simulink model "manualControl"  (R2019a)
settings: Solver=FixedStepDiscrete  StartTime=0.0  StopTime=60  FixedStep=0.1  RelTol=1e-3  EnableMultiTasking=on
model workspace (MAT data in the model file):
  SL_ROS_VariableLengthArrays_MaxSizes.CommonInfo.ArrayTruncateAction = 'EmitWarning'
  SL_ROS_VariableLengthArrays_MaxSizes.MsgTypeMap = containers.Map
  SL_ROS_VariableLengthArrays_MaxSizes.MsgTypeMap.serialization.keys = {'sensor_msgs/Image', 'sensor_msgs/LaserScan'}
  SL_ROS_VariableLengthArrays_MaxSizes.MsgTypeMap.serialization.values{1}(1).PropertyName = 'Data'
  SL_ROS_VariableLengthArrays_MaxSizes.MsgTypeMap.serialization.values{1}(1).DataType = 'uint8'
  SL_ROS_VariableLengthArrays_MaxSizes.MsgTypeMap.serialization.values{1}(1).MaxLength = 691200
  SL_ROS_VariableLengthArrays_MaxSizes.MsgTypeMap.serialization.values{1}(2).PropertyName = 'Encoding'
  SL_ROS_VariableLengthArrays_MaxSizes.MsgTypeMap.serialization.values{1}(2).DataType = 'uint8'
  SL_ROS_VariableLengthArrays_MaxSizes.MsgTypeMap.serialization.values{1}(2).MaxLength = 128
  SL_ROS_VariableLengthArrays_MaxSizes.MsgTypeMap.serialization.values{2}(1).PropertyName = 'Intensities'
  SL_ROS_VariableLengthArrays_MaxSizes.MsgTypeMap.serialization.values{2}(1).DataType = 'single'
  SL_ROS_VariableLengthArrays_MaxSizes.MsgTypeMap.serialization.values{2}(1).MaxLength = 1081
  SL_ROS_VariableLengthArrays_MaxSizes.MsgTypeMap.serialization.values{2}(2).PropertyName = 'Ranges'
  SL_ROS_VariableLengthArrays_MaxSizes.MsgTypeMap.serialization.values{2}(2).DataType = 'single'
  SL_ROS_VariableLengthArrays_MaxSizes.MsgTypeMap.serialization.values{2}(2).MaxLength = 1081
  SL_ROS_VariableLengthArrays_MaxSizes.MsgTypeMap.serialization.uniformity = 0
  SL_ROS_VariableLengthArrays_MaxSizes.MsgTypeMap.serialization.keyType = 'char'
  SL_ROS_VariableLengthArrays_MaxSizes.MsgTypeMap.serialization.valueType = 'any'
undefined symbols (not defined in the file or in its folder): Angular, d, dfod, DiscIntNeverNeededParam, gray, ioKd, ioKi, ioKp, Kd, Kp, Linear
libraries: robotlib x6, simulink x2, aerolibanimutils x1
settings Model: Creator=The MathWorks, Inc.  LastModifiedBy=standard
settings DataIOCC: LimitDataPoints=on  SaveFormat=Array  ReturnWorkspaceOutputs=off
settings OptimizationCC: LifeSpan=Inf  MaxStackSize=64
settings DebuggingCC: SolverPrmCheckMsg=warning  SFUnexpectedBacktrackingDiag=warning  SFNoUnconditionalDefaultTransitionDiag=warning  SFExecutionAtInitializationDiag=none  ArithmeticOperatorsInVariantConditions=warning
settings HardwareCC: ProdBitPerPointer=32  ProdBitPerSizeT=32  ProdBitPerPtrDiffT=32  ProdLargestAtomicFloat=None  ProdIntDivRoundTo=Undefined  ProdEndianess=Unspecified  ProdWordSize=32  ProdHWDeviceType=Generic->Unspecified (assume 32-bit Generic)  UseEmbeddedCoderFeatures=off
settings ModelReferenceCC: PropagateSignalLabelsOutOfModel=off
settings SFSimCC: SimUseLocalCustomCode=off
settings RTWCC: SystemTargetFile=ert.tlc  HardwareBoard=Robot Operating System (ROS)  TLCOptions=-aInlineSetEventsForThisBaseRateFcn=TLC_FALSE -aSuppressMultiTaskScheduler=TLC_FALSE -aRateBasedStepFcn=0  TemplateMakefile=ert_default_tmf  RTWUseLocalCustomCode=off  Toolchain=Catkin  TargetLang=C++
settings CodeAppCC: StateflowObjectComments=on
settings ERTTargetCC: MultiwordLength=2048  ERTCustomFileBanners=off  SupportContinuousTime=on  SupportNonInlinedSFcns=on  RemoveResetFunc=off  SupportVariableSizeSignals=on  ModelStepFunctionPrototypeControlCompliant=off  ConvertIfToSwitch=off  SuppressUnreachableDefaultCases=off
settings ConfigComp: CovMetricSettings=dw  CovHtmlReporting=on  CovSaveCumulativeToWorkspaceVar=on  CovSaveSingleToWorkspaceVar=on  CovExternalEMLEnable=off  CovSFcnEnable=off

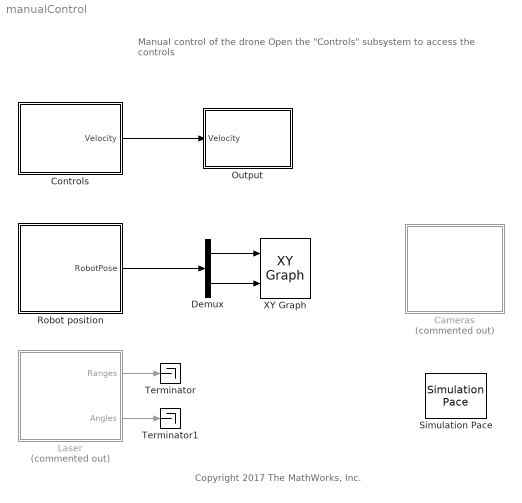
== system manualControl ==
  note: Manual control of the drone
      | Open the "Controls" subsystem to access the controls
  note: Copyright 2017 The MathWorks, Inc.
  Cameras : Subsystem  Commented=on
  Controls : Subsystem
  Demux : Demux  Outputs=2
  Laser : Subsystem  Commented=on
  Output : Subsystem
  Robot position : Subsystem
  Simulation Pace : aerolibanimutils/Simulation Pace  SimulationPace=1  SleepMode=MATLAB Thread  OutputPaceError=off  SampleTime=-1
  Terminator : Terminator
  Terminator1 : Terminator
  XY Graph : simulink/Sinks/XY Graph  xmin=-10  xmax=30  ymin=-10  ymax=10  st=-1
  wires:
  Controls/1(Velocity) -> Output/1(Velocity)
  Robot position/1(RobotPose) -> Demux/1
  Demux/1 -> XY Graph/1
  Demux/2 -> XY Graph/2
  Laser/1(Ranges) -> Terminator/1
  Laser/2(Angles) -> Terminator1/1

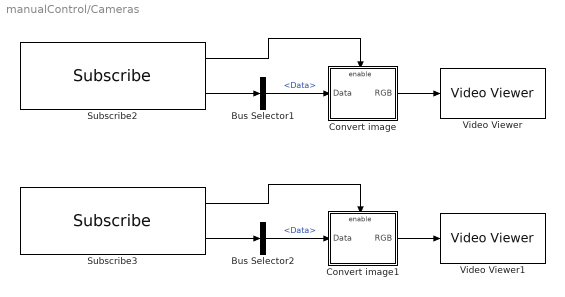
== system manualControl/Cameras ==
  Bus Selector1 : BusSelector  DialogController=Simulink.DDGSource_BusSelector  OutputSignals=Data
  Bus Selector2 : BusSelector  DialogController=Simulink.DDGSource_BusSelector  OutputSignals=Data
  Convert image : Subsystem
  Convert image1 : Subsystem
  Subscribe2 : robotlib/Subscribe  topicSource=Select from ROS network  topic=/quadrotor_1/front/image_raw  messageType=sensor_msgs/Image  sampleTime=-1  messageQueueLength=51
      settings: SourceProductBaseCode=RO
  Subscribe3 : robotlib/Subscribe  topicSource=Select from ROS network  topic=/quadrotor_1/bottom/image_raw  messageType=sensor_msgs/Image  sampleTime=-1  messageQueueLength=51
      settings: SourceProductBaseCode=RO
  Video Viewer : VideoViewer  colormapValue=gray(256)  FigPos=[672 404 609 271.6]
  Video Viewer1 : VideoViewer  colormapValue=gray(256)  FigPos=[671 757 610 376]
  wires:
  Subscribe2/1 -> Convert image/Enable
  Convert image1/1(RGB) -> Video Viewer1/1
  Subscribe3/2 -> Bus Selector2/1
  Subscribe2/2 -> Bus Selector1/1
  Bus Selector1/1 -> Convert image/1(Data)  "<Data>"
  Bus Selector2/1 -> Convert image1/1(Data)  "<Data>"
  Subscribe3/1 -> Convert image1/Enable
  Convert image/1(RGB) -> Video Viewer/1

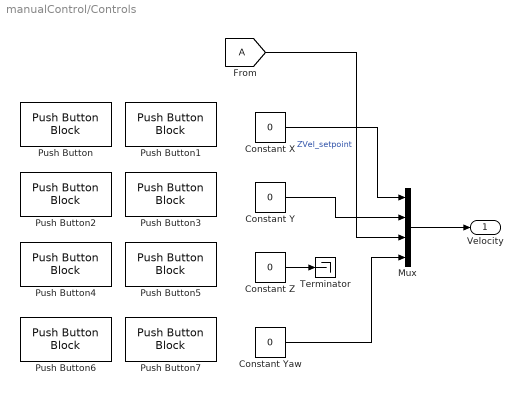
== system manualControl/Controls ==
  Constant X : Constant  Value=0
  Constant Y : Constant  Value=0
  Constant Yaw : Constant  Value=0
  Constant Z : Constant  Value=0
  Mux : Mux
  Push Button : PushButtonBlock  LabelPosition=Top  ButtonText=Backward  OnValue=-1
  Push Button1 : PushButtonBlock  LabelPosition=Top  ButtonText=Forward
  Push Button2 : PushButtonBlock  LabelPosition=Top  ButtonText=Left
  Push Button3 : PushButtonBlock  LabelPosition=Top  ButtonText=Right  OnValue=-1
  Push Button4 : PushButtonBlock  LabelPosition=Top  ButtonText=Down  OnValue=-1
  Push Button5 : PushButtonBlock  LabelPosition=Top  ButtonText=Up
  Push Button6 : PushButtonBlock  LabelPosition=Top  ButtonText=Counterclockwise
  Push Button7 : PushButtonBlock  LabelPosition=Top  ButtonText=Clockwise  OnValue=-1
  Terminator : Terminator
  Velocity : Outport
  wires:
  Mux/1 -> Velocity/1
  Constant Y/1 -> Mux/2
  Constant X/1 -> Mux/1
  [A] -> Mux/3  "ZVel_setpoint"
  Constant Yaw/1 -> Mux/4
  Constant Z/1 -> Terminator/1

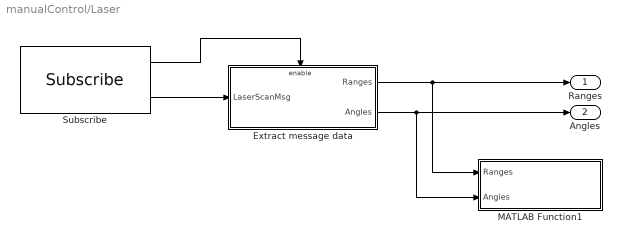
== system manualControl/Laser ==
  Extract message data : Subsystem
  MATLAB Function1 : MATLAB Function  TreatAsAtomicUnit=on
  Subscribe : robotlib/Subscribe  topicSource=Select from ROS network  topic=/quadrotor_1/scan  messageType=sensor_msgs/LaserScan  sampleTime=-1  messageQueueLength=1
      settings: SourceProductBaseCode=RO
  Ranges : Outport
  Angles : Outport  Port=2
  wires:
  Subscribe/1 -> Extract message data/Enable
  Extract message data/2(Angles) -> Angles/1, MATLAB Function1/2(Angles)
  Subscribe/2 -> Extract message data/1(LaserScanMsg)
  Extract message data/1(Ranges) -> Ranges/1, MATLAB Function1/1(Ranges)

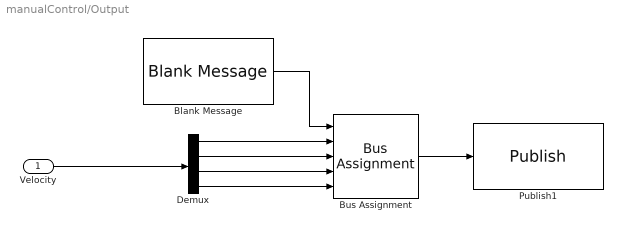
== system manualControl/Output ==
  Velocity : Inport
  Blank Message : robotlib/Blank Message  messageClass=Message  entityType=geometry_msgs/Twist  messageType=geometry_msgs/Twist  SampleTime=0
      settings: SourceProductBaseCode=RO
  Bus Assignment : BusAssignment  DialogController=Simulink.DDGSource_BusAssignment  AssignedSignals=Linear.X,Linear.Y,Linear.Z,Angular.Z
  Demux : Demux
  Publish1 : robotlib/Publish  topicSource=Select from ROS network  topic=/quadrotor_1/cmd_vel  messageType=geometry_msgs/Twist  messageQueueLength=105
      settings: SourceProductBaseCode=RO
  wires:
  Demux/2 -> Bus Assignment/3
  Demux/1 -> Bus Assignment/2
  Demux/3 -> Bus Assignment/4
  Demux/4 -> Bus Assignment/5
  Velocity/1 -> Demux/1
  Bus Assignment/1 -> Publish1/1
  Blank Message/1 -> Bus Assignment/1

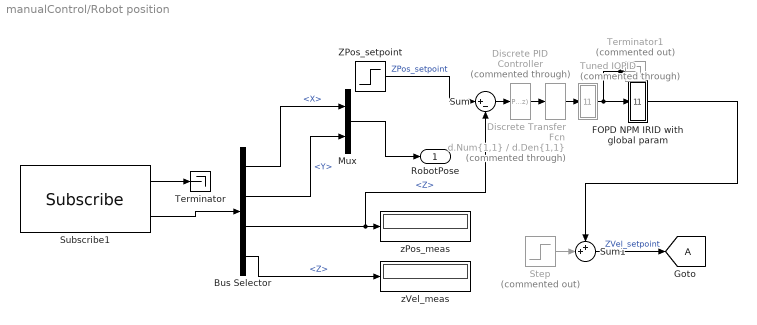
== system manualControl/Robot position ==
  Bus Selector : BusSelector  DialogController=Simulink.DDGSource_BusSelector  OutputSignals=Pose.Pose.Position.X,Pose.Pose.Position.Y,Pose.Pose.Position.Z,Twist.Twist.Linear.Z
  Discrete Transfer Fcn : DiscreteTransferFcn  Commented=through  Numerator=d.Num{1,1}  Denominator=d.Den{1,1}
  Discrete PID Controller : simulink/Continuous/PID Controller  Commented=through  Controller=PID  Form=Parallel  TimeDomain=Discrete-time  SampleTime=-1  IntegratorMethod=Forward Euler  FilterMethod=Forward Euler  ControllerParametersSource=internal  P=4  I=0  D=0  UseFilter=on  N=100  TunerSelectOption=Transfer Function Based (PID Tuner App)  InitialConditionSource=internal  InitialConditionForIntegrator=0  InitialConditionForFilter=0  DifferentiatorICPrevScaledInput=0  ExternalReset=none  TrackingMode=off  Kt=1  LimitOutput=on  UpperSaturationLimit=inf  LowerSaturationLimit=-inf  LinearizeAsGain=off  AntiWindupMode=back-calculation  Kb=1  POutMin=[]  POutMax=[]  IOutMin=[]  IOutMax=[]  DOutMin=[]  DOutMax=[]  NOutMin=[]  NOutMax=[]  SumOutMin=[]  SumOutMax=[]  SaturationOutMin=[]  SaturationOutMax=[]  PParamMin=[]  PParamMax=[]  IParamMin=[]  IParamMax=[]  DParamMin=[]  DParamMax=[]  NParamMin=[]  NParamMax=[]  KbParamMin=[]  KbParamMax=[]  KtParamMin=[]  KtParamMax=[]  KbOutMin=[]  KbOutMax=[]  KtOutMin=[]  KtOutMax=[]  IntegratorOutMin=[]  IntegratorOutMax=[]  FilterOutMin=[]  FilterOutMax=[]  SumI1OutMin=[]  SumI1OutMax=[]  SumI2OutMin=[]  SumI2OutMax=[]  SumI3OutMin=[]  SumI3OutMax=[]  SumI4OutMin=[]  SumI4OutMax=[]  SumDOutMin=[]  SumDOutMax=[]  DifferentiatorOutMin=[]  DifferentiatorOutMax=[]  FilterDiffOutCoefMin=[]  FilterDiffOutCoefMax=[]  ReciprocalOutMin=[]  ReciprocalOutMax=[]  SumDenOutMin=[]  SumDenOutMax=[]  SumNumOutMin=[]  SumNumOutMax=[]  DivideOutMin=[]  DivideOutMax=[]  IntegratorContinuousStateAttributes=''  IntegratorStateMustResolveToSignalObject=off  IntegratorRTWStateStorageClass=Auto  FilterContinuousStateAttributes=''  FilterStateMustResolveToSignalObject=off  FilterRTWStateStorageClass=Auto  ParallelPVariant=InternalParameters  IdealPVariant=Disabled  IVariant=InternalParameters  DVariant=InternalParameters  IntegratorVariant=Discrete  SatVariant=Enabled  AWVariant=BackCalculation  PCopyVariant=Disabled  TRVariant=Disabled  FdbkBlocksVariant=Forward  IdealPFdbkVariant=Disabled  SatFdbkVariant=Disabled  DerivativeFilterVariant=ForwardEulerFilter  NVariant=InternalParameters  NCopyVariant=Disabled  FilterICVariant=InternalICsFilter  IntegratorICVariant=InternalICs  ExternalResetVariant=Disabled  TRSumVariant=Passthrough  SumFdbkVariant=Disabled  SumVariant=Sum_PID
  FOPD NPM IRID with global param : Subsystem
  Mux : Mux  Inputs=2
  Step : Step  Commented=on  Time=5  SampleTime=0.1
  Subscribe1 : robotlib/Subscribe  topicSource=Select from ROS network  topic=/quadrotor_1/ground_truth/state  messageType=nav_msgs/Odometry  sampleTime=-1  messageQueueLength=51
      settings: SourceProductBaseCode=RO
  Sum : Sum  Inputs=|+-
  Sum1 : Sum  Inputs=++|
  Terminator : Terminator
  Terminator1 : Terminator  Commented=on
  Tuned IOPID : Subsystem  Commented=through
  ZPos_setpoint : Step  Time=10  SampleTime=0.1
  zPos_meas : Display
  zVel_meas : Display
  RobotPose : Outport
  tag scope: A=global
  wires:
  Subscribe1/2 -> Bus Selector/1
  Subscribe1/1 -> Terminator/1
  Bus Selector/1 -> Mux/1  "<X>"
  Bus Selector/2 -> Mux/2  "<Y>"
  Mux/1 -> RobotPose/1
  Bus Selector/3 -> Sum/2, zPos_meas/1  "<Z>"
  Bus Selector/4 -> zVel_meas/1  "<Z>"
  ZPos_setpoint/1 -> Sum/1  "ZPos_setpoint"
  Sum/1 -> Discrete PID Controller/1
  Discrete PID Controller/1 -> Discrete Transfer Fcn/1
  Sum1/1 -> [A]  "ZVel_setpoint"
  FOPD NPM IRID with global param/1(Out1) -> Sum1/1
  Step/1 -> Sum1/2
  Tuned IOPID/1(Out1) -> FOPD NPM IRID with global param/1(In1), Terminator1/1
  Discrete Transfer Fcn/1 -> Tuned IOPID/1(In1)

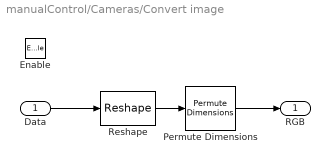
== system manualControl/Cameras/Convert image ==
  Data : Inport
  Enable : EnablePort
  Permute Dimensions : PermuteDimensions  Order=[3 2 1]
  Reshape : Reshape  OutputDimensionality=Customize  OutputDimensions=[3 640 360]
  RGB : Outport
  wires:
  Permute Dimensions/1 -> RGB/1
  Reshape/1 -> Permute Dimensions/1
  Data/1 -> Reshape/1

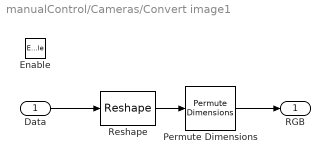
== system manualControl/Cameras/Convert image1 ==
  Data : Inport
  Enable : EnablePort
  Permute Dimensions : PermuteDimensions  Order=[3 2 1]
  Reshape : Reshape  OutputDimensionality=Customize  OutputDimensions=[3 640 360]
  RGB : Outport
  wires:
  Permute Dimensions/1 -> RGB/1
  Reshape/1 -> Permute Dimensions/1
  Data/1 -> Reshape/1

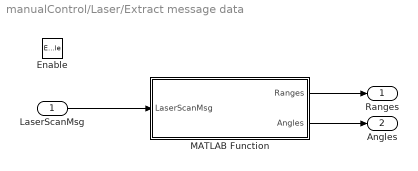
== system manualControl/Laser/Extract message data ==
  LaserScanMsg : Inport
  Enable : EnablePort
  MATLAB Function : MATLAB Function  TreatAsAtomicUnit=on
  Ranges : Outport
  Angles : Outport  Port=2
  wires:
  MATLAB Function/1(Ranges) -> Ranges/1
  MATLAB Function/2(Angles) -> Angles/1
  LaserScanMsg/1 -> MATLAB Function/1(LaserScanMsg)

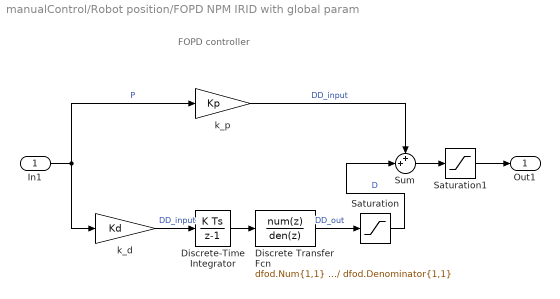
== system manualControl/Robot position/FOPD NPM IRID with global param ==
  note: FOPD controller
  In1 : Inport
  Discrete Transfer Fcn : DiscreteTransferFcn  Numerator=dfod.Num{1,1}  Denominator=dfod.Denominator{1,1}  SampleTime=0.1
  Discrete-Time Integrator : DiscreteIntegrator  SampleTime=0.1  ICPrevOutput=DiscIntNeverNeededParam  ICPrevScaledInput=DiscIntNeverNeededParam
  Saturation : Saturate  UpperLimit=100  LowerLimit=-100
  Saturation1 : Saturate  UpperLimit=200  LowerLimit=-200
  Sum : Sum  Inputs=++|
  k_d : Gain  Gain=Kd
  k_p : Gain  Gain=Kp
  Out1 : Outport
  wires:
  In1/1 -> k_p/1, k_d/1  "P"
  Sum/1 -> Saturation1/1
  Saturation1/1 -> Out1/1
  k_p/1 -> Sum/1  "DD_input"
  k_d/1 -> Discrete-Time Integrator/1  "DD_input"
  Discrete Transfer Fcn/1 -> Saturation/1  "DD_out"
  Saturation/1 -> Sum/2  "D"
  Discrete-Time Integrator/1 -> Discrete Transfer Fcn/1

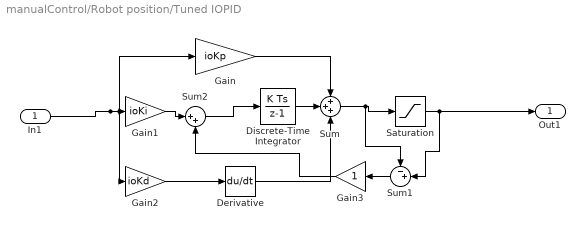
== system manualControl/Robot position/Tuned IOPID ==
  In1 : Inport
  Derivative : Derivative
  Discrete-Time Integrator : DiscreteIntegrator  SampleTime=-1  ICPrevOutput=DiscIntNeverNeededParam  ICPrevScaledInput=DiscIntNeverNeededParam
  Gain : Gain  Gain=ioKp
  Gain1 : Gain  Gain=ioKi
  Gain2 : Gain  Gain=ioKd
  Gain3 : Gain
  Saturation : Saturate  UpperLimit=10  LowerLimit=-10
  Sum : Sum  Inputs=+++
  Sum1 : Sum  Inputs=-+|
  Sum2 : Sum  Inputs=|++
  Out1 : Outport
  wires:
  Sum/1 -> Sum1/1, Saturation/1
  Sum1/1 -> Gain3/1
  In1/1 -> Gain2/1, Gain/1, Gain1/1
  Sum2/1 -> Discrete-Time Integrator/1
  Derivative/1 -> Sum/3
  Gain/1 -> Sum/1
  Discrete-Time Integrator/1 -> Sum/2
  Gain1/1 -> Sum2/1
  Gain3/1 -> Sum2/2
  Gain2/1 -> Derivative/1
  Saturation/1 -> Sum1/2, Out1/1

== matlab function manualControl/Laser/MATLAB Function1 ==
  data: Ranges input; Angles input
function plotLaser(Ranges, Angles)
coder.extrinsic('polarplot');
persistent p;
if isempty(p)
    p = polarplot(0, 0, '.');
    set(gca, 'ThetaZeroLocation', 'top', 'ThetaLim', [-135 135], ...
        'RAxisLocation', 0, 'RLim', [0 10]);
end
if ishandle(p)
    set(p, 'ThetaData', Angles);
    set(p, 'RData', Ranges);
    drawnow limitrate;
end

== matlab function manualControl/Laser/Extract message data/MATLAB Function ==
  data: LaserScanMsg input; Ranges output size=[1081 1]; Angles output size=[1081 1]
function [Ranges, Angles] = ExtractRangeData(LaserScanMsg)
%#codegen

% Extract Range information
Ranges = double(LaserScanMsg.Ranges);

% Construct Angles vector using AngleMin and AngleIncrement from sensor
% reading.
angMin = double(LaserScanMsg.AngleMin);
angMax = double(LaserScanMsg.AngleMax);
rawAngles = linspace(angMax, angMin, numel(Ranges)).';

% Wrap the angles to the (-pi,pi] interval.
Angles = robotics.internal.wrapToPi(double(rawAngles));
